simulink library "SUB_L4_Task_100ms"  (R2018a)
settings: Solver=VariableStepAuto  StartTime=0.0  StopTime=10.0  RelTol=1e-3
settings Model: Creator=Chris.Balton  LastModifiedBy=Chris.Balton

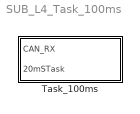
== system SUB_L4_Task_100ms ==
  Task_100ms : Subsystem  TreatAsAtomicUnit=on  SystemSampleTime=0.1

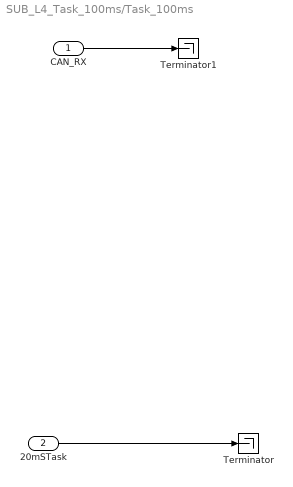
== system SUB_L4_Task_100ms/Task_100ms ==
  CAN_RX : Inport
  20mSTask : Inport  Port=2
  Terminator : Terminator
  Terminator1 : Terminator
  wires:
  20mSTask/1 -> Terminator/1
  CAN_RX/1 -> Terminator1/1
